simulink library "DAEMOT_Lib"  (R2019b)
settings: Solver=ode45  StartTime=0.0  StopTime=10.0  FixedStep=0.1  RelTol=1e-3
undefined symbols (not defined in the file or in its folder): Controller, CP, Ctrl, Ctrl_Fcn, Elec1, f, F2, Fluid, lag1, Mission, Moody, PropellerProp, rev_comms_sink
libraries: $bdroot x200, instrumentlib x21, simulink x5, dspsigops x2
(part 6 of 13)

== system DAEMOT_Lib/Thermal ==
  Air Volume : Subsystem  mask(Air volume){fld=Air, T_init=22, M_init=262.8177, P_init=105, Tamb_init=22, H=0, D=3, L=30, V=212.0575, A_sa=282.7433, Pamb=101, E_fluid=101*1e3}
      mask prompts: fld "Fluid Type"; T_init "Initial Air Temperature [°C]"; M_init "Initial Fluid Mass [kg]"; P_init "Air Pressure [kPa]"; Tamb_init "Initial Ambient Temperature [°C]"; H "Heat Transfer Coefficient with Ambient [W/m²K]"; D "Air Volume Diameter [m]"; L "Air Volume Length [m]"; V "Air Volume [m³]"; A_sa "Air Volume Surface Area [m²]"; Pamb "Ambient Pressure [kPa]"; E_fluid "Bulk Modulus"
      mask help: Tracks the time rate of change for fluid mass and temperature.
      mask init:
      | load('Fluids.mat');
      | Fluid = eval(['Fluid.',fld]);
      | 
      | % calculate the volume -- assuming a cylinder
      | V = L*pi*D^2/4;    
      | set_param(gcb,'V',num2str(V));
      | 
      | % calculate the surface area -- assuming a cylinder
      | SA = L * pi * D ;
      | set_param(gcb,'A_sa',num2str(SA));
      | 
      | % Note: Assumes a fixed initial pressure to calculate density
      | P_for_rho = 105;
      | Rho = qminterp2(Fluid.T, Fluid.P, Fluid.Rho_pt, T_init, P_for_rho);
      | 
      | % set the mass of air in the air volume
      | set_param(gcb,'M_init',num2str(Rho*V));
      settings: OpenFcn=|
      | load('Fluids.mat');
      | Set_Fluid_Popup_Names( Fluid )
      mask TypeOptions fld: Fuel | Water | Air | PG50
      mask DialogControl Container8 Prompt: Parameters
      mask DialogControl Container10 Prompt: Nonlinear Model
      mask DialogControl NomValuesGroupVar Prompt: Component Sizing - Nominal Values
      mask DialogControl Container11 Prompt: Linear Model
      mask Display:
      | image(imread('cabin.png'))
      | 
      | text(0.5,0.9,['{\bf Air Volume}'],'TexMode','on','horizontalAlignment', 'center')
      | text(0.5,0.1,['{(P)}'],'TexMode','on','horizontalAlignment', 'center')
      | 
      | port_label('input',1,'Flow In')
      | port_label('input',2,'Amb. Temp. [°C]')
      | port_label('input',3,'Q internal [kW]')
      | port_label('output',1,'Flow Out')
      | % port_label('output',2,'Fluid Mass [kg]')
  Cold_Plate : Subsystem  mask(Cold Plate){fld=PG50, P_init=113, Tw_init=20, T_init=20, f=0.035, KL=0, PAF=1, HTC_method=on, HTC=4000, M_wall=1, Cp_wall=0.9, D=0.03, L=1.5, t=0.0015, E=2.4e6, v=0.4, dH=0, e_rough=CP.e*1e-3}
      mask prompts: fld "Fluid Type"; P_init "Initial Outlet Pressure [kPa]"; Tw_init "Initial Wall Temperature [°C]"; T_init "Initial Outlet Temperature [°C]"; f "Friction Factor [-]"; KL "Minor Losses [-]"; PAF "HTC Parameter Adjustment Factor [-]"; HTC_method "User-Defined Heat Transfer Coefficient?"; HTC "Heat Transfer Coefficient [W/m^2*K]"; M_wall "Wall Mass [kg]"; Cp_wall "Wall Specific Heat [kJ/kg*K]"; D "Internal Diameter [m]"; L "Tube Length [m]"; t "Tube Wall Thickness [m]"; E "Tube Modulus of Elasticity [kPa]"; v "Tube Poisson Ratio [-]"; dH "Height between Inlet and Outlet [m]"; e_rough "Surface Roughness [m] (0.0015mm for copper, 0.01mm for rubber, 0mm for plastic)"
      mask help: Tracks the time rate of change of the pressure, wall temperature, and fluid exit temperature.
      mask init:
      | load('Fluids.mat');
      | Fluid = eval(['Fluid.',fld]);
      | 
      | load('Moody.mat');
      settings: OpenFcn=|
      | load('Fluids.mat');
      | Set_Fluid_Popup_Names( Fluid )
      mask TypeOptions fld: Fuel | Water | Air | PG50
      mask Callback HTC_method:
      | en = get_param(gcb,'MaskVisibilities');
      | 
      | switch get_param(gcb,'HTC_method')
      |     case 'on'
      |         en{9} = 'on';
      |     case 'off'
      |         en{9} = 'off';
      | end
      | set_param(gcb,'MaskVisibilities',en);
      mask DialogControl Container5 Prompt: Parameters
      mask DialogControl Container8 Prompt: Nonlinear Model
      mask DialogControl Container13 Prompt: Component Sizing - Nominal Values
      mask DialogControl Container11 Prompt: Linear Model
      mask Display:
      | image(imread('ColdPlate.jpg'))
      | 
      | text(0.5,0.95,['{\bf ',fld,' Cold Plate}'],'TexMode','on','horizontalAlignment', 'center')
      | text(0.5,0.08,['{-----(P)}'],'TexMode','on','horizontalAlignment', 'center')
      | 
      | port_label('input',1,'Flow In')
      | port_label('input',2,'Thermal In')
      | port_label('output',1,'Flow Out')
  Flow Split_Junction : Subsystem  mask(Split/Junction){fld=PG50, Num_Out=1, Num_In=1, P_init=110, T_init=22, D=0.013, L=0.1, t=0.0015, E=2.4e6, v=0.4}
      mask prompts: fld "Fluid Type"; Num_Out "Number of Outlet Flows"; Num_In "Number of Inlet Flows"; P_init "Initial Pressure [kPa]"; T_init "Initial Temperature [°C]"; D "Diameter [m]"; L "Length [m]"; t "Tube Wall Thickness [m]"; E "Tube Modulus of Elasticity [kPa]"; v "Tube Poisson Ratio [-]"
      mask help: Splits and junctions flows using dynamic relationships. Note that the library link of the block is disabled when it is imported into a model.
      mask init:
      | h      = get_param(gcb,'handle');   % Get block handle
      | blk    = gcb;
      | hblock = get(h);     % Parse out handles structure
      | 
      | load('Fluids.mat');
      | Fluid = eval(['Fluid.',fld]);
      | 
      | % delete any previous inports and bus selectors
      | for i = str2num(hblock.Num_In)+1:hblock.Ports(1)
      |     delete_block([blk,'/In',num2str(i)])
      |     delete_block([blk,'/gb',num2str(i)])
      |     delete_block([blk,'/gm',num2str(i)])
      |     delete_block([blk,'/gt',num2str(i)])
      |     delete_block([blk,'/gp',num2str(i)])
      |     delete_block([blk,'/Sink',num2str(i)])
      |     delete_block([blk,'/pout',num2str(i)])
      |     delete_block([blk,'/min',num2str(i)])
      |     delete_block([blk,'/tin',num2str(i)])
      |     
      |     delete_unconnected_lines(blk)
      | end
      | 
      | % delete any previous inports and bus selectors
      | for i = str2num(hblock.Num_Out)+1:hblock.Ports(2)
      |     delete_block([blk,'/Out',num2str(i)])
      |     delete_block([blk,'/m',num2str(i)])
      |     delete_block([blk,'/t',num2str(i)])
      |     delete_block([blk,'/p',num2str(i)])
      |     delete_block([blk,'/b',num2str(i)])
      |     delete_block([blk,'/Source',num2str(i)])
      |     delete_block([blk,'/g',num2str(i)])
      |     delete_block([blk,'/mout',num2str(i)])
      |     %delete_block([blk,'/tout',num2str(i)])
      |     
      |     delete_unconnected_lines(blk)
      | end
      | 
      | set_param([blk,'/Mux_In_1'],'Inputs',hblock.Num_In)
      | set_param([blk,'/Mux_In_2'],'Inputs',hblock.Num_Out)
      | set_param([blk,'/Mux_In_3'],'Inputs',hblock.Num_In)
      | %set_param([blk,'/Mux_Out_1'],'Outputs',hblock.Num_Out)
      | 
      | % generate inports, bus selectors, and route lines to each vector concat
      | for i = hblock.Ports(1)+1:str2num(hblock.Num_In)
      |     
      |     % add blocks
      |     add_block('simulink/Ports & Subsystems/In1',   [blk,'/In',num2str(i)],    'Position',[120 i*80-25+20 150 i*80-12+20]);         % adding inport
      |     add_block([blk,'/gb1'],                        [blk,'/gb',num2str(i)],   'Position',[200 i*80-20+20-18 205 i*80-2+20+2]);         % adding inport
      |     add_block('simulink/Signal Routing/Goto',      [blk,'/gm',num2str(i)],    'Position',[260 i*80-17 340 i*80-3]);         % adding inport
      |     add_block('simulink/Signal Routing/Goto',      [blk,'/gt',num2str(i)],    'Position',[260 i*80+3 340 i*80+17]);         % adding inport
      |     add_block('simulink/Sinks/Terminator',          [blk,'/gp',num2str(i)],    'Position',[260 i*80+23 280 i*80+37]);         % adding inport
      |     add_block('DAEMOT_Lib/Support Functions/Sink',[blk,'/Sink',num2str(i)],'Position',[745 i*80-14 810 i*80+14]);         % adding inport
      |     add_block('simulink/Signal Routing/From',      [blk,'/pout',num2str(i)],    'Position',[625 i*80-14 705 i*80+14]);         % adding inport
      |     add_block('simulink/Signal Routing/From',       [blk,'/min',num2str(i)],     'Position',[935 -258+i*20 1015 -242+i*20]);         % adding inport
      |     add_block('simulink/Signal Routing/From',       [blk,'/tin',num2str(i)],     'Position',[935 1+i*20 1015 19+i*20]);         % adding inport
      |     
      |     % set goto and from tags
      |     set_param([blk,'/gm',num2str(i)],'GotoTag',char(horzcat('M_in',num2str(i))))
      |     set_param([blk,'/gt',num2str(i)],'GotoTag',char(horzcat('T_in',num2str(i))))
      |     %set_param([blk,'/gp',num2str(i)],'GotoTag',char(horzcat('P_in',num2str(i))))
      |     set_param([blk,'/pout',num2str(i)],'GotoTag',char('P'))
      |     set_param([blk,'/min',num2str(i)],'GotoTag',char(horzcat('M_in',num2str(i))))
      |     set_param([blk,'/tin',num2str(i)],'GotoTag',char(horzcat('T_in',num2str(i))))
      |     
      |     % set goto and from background colors
      |     set_param([blk,'/gm',num2str(i)],'BackgroundColor','yellow')
      |     set_param([blk,'/gt',num2str(i)],'BackgroundColor','yellow')
      |     %set_param([blk,'/gp',num2str(i)],'BackgroundColor','yellow')
      |     set_param([blk,'/min',num2str(i)],'BackgroundColor','yellow')
      |     set_param([blk,'/tin',num2str(i)],'BackgroundColor','yellow')
      |     set_param([blk,'/pout',num2str(i)],'BackgroundColor','cyan')
      |     
      |     % add lines
      |     add_line(blk,['In',num2str(i),'/1'], ['gb',num2str(i),'/1'],'AutoRouting','on')
      |     add_line(blk,['gb',num2str(i),'/1'],  ['gm',num2str(i),'/1'],'AutoRouting','on')
      |     add_line(blk,['gb',num2str(i),'/2'],  ['gt',num2str(i),'/1'],'AutoRouting','on')
      |     add_line(blk,['gb',num2str(i),'/3'],  ['gp',num2str(i),'/1'],'AutoRouting','on')
      |     add_line(blk,['pout',num2str(i),'/1'],  ['Sink',num2str(i),'/1'],'AutoRouting','on')
      |     add_line(blk,['min',num2str(i),'/1'],  ['Mux_In_1/',num2str(i)],'AutoRouting','on')
      |     add_line(blk,['tin',num2str(i),'/1'],  ['Mux_In_3/',num2str(i)],'AutoRouting','on')
      |     
      | end
      | 
      | % generate inports, bus selectors, and route lines to each vector concat
      | for i = hblock.Ports(2)+1:str2num(hblock.Num_Out)
      |     
      |     % add blocks
      |     add_block('simulink/Ports & Subsystems/Out1',   [blk,'/Out',num2str(i)],   'Position',[30 i*80-25+20 60 i*80-12+20]);         % adding inport
      |     add_block('simulink/Signal Routing/From',       [blk,'/m',num2str(i)],     'Position',[-150 i*80-20 -70 i*80-2]);         % adding inport
      |     add_block('simulink/Signal Routing/From',       [blk,'/t',num2str(i)],     'Position',[-150 i*80-20+20 -70 i*80-2+20]);         % adding inport
      |     add_block('simulink/Signal Routing/From',       [blk,'/p',num2str(i)],     'Position',[-150 i*80-20+40 -70 i*80-2+40]);         % adding inport
      |     add_block('simulink/Signal Routing/Bus Creator',[blk,'/b',num2str(i)],     'Position',[5 i*80-20+20-18 10 i*80-2+20+2]);         % adding inport
      |     add_block('DAEMOT_Lib/Support Functions/Source',[blk,'/Source',num2str(i)],'Position',[395 i*80-14 460 i*80+14]);         % adding inport
      |     add_block('simulink/Signal Routing/Goto',       [blk,'/g',num2str(i)],     'Position',[505 i*80-9 585 i*80+9]);         % adding inport
      |     add_block('simulink/Signal Routing/From',       [blk,'/mout',num2str(i)],  'Position',[935 -129+i*20 1015 -111+i*20]);         % adding inport
      |     %add_block('simulink/Signal Routing/Goto',      [blk,'/tout',num2str(i)],   'Position',[1455 -259+i*20 1535 -241+i*20]);         % adding inport
      |     
      |     % set goto and from tags
      |     set_param([blk,'/m',num2str(i)],'GotoTag',char(horzcat('M_out',num2str(i))))
      |     %set_param([blk,'/t',num2str(i)],'GotoTag',char(horzcat('T_out',num2str(i))))
      |     set_param([blk,'/t',num2str(i)],'GotoTag',char('T'))
      |     set_param([blk,'/p',num2str(i)],'GotoTag',char('P'))
      |     set_param([blk,'/g',num2str(i)],'GotoTag',char(horzcat('M_out',num2str(i))))
      |     set_param([blk,'/mout',num2str(i)],'GotoTag',char(horzcat('M_out',num2str(i))))
      |     %set_param([blk,'/tout',num2str(i)],'GotoTag',char(horzcat('T_out',num2str(i))))
      |     set_param([blk,'/b',num2str(i)],'Inputs','3')
      |     
      |     % set goto and from background colors
      |     set_param([blk,'/t',num2str(i)],'BackgroundColor','cyan')
      |     set_param([blk,'/m',num2str(i)],'BackgroundColor','cyan')
      |     set_param([blk,'/p',num2str(i)],'BackgroundColor','cyan')
      |     set_param([blk,'/g',num2str(i)],'BackgroundColor','cyan')
      |     set_param([blk,'/mout',num2str(i)],'BackgroundColor','cyan')
      |     %set_param([blk,'/tout',num2str(i)],'BackgroundColor','cyan')
      |     
      |     % add lines
      |     add_line(blk,['m',num2str(i),'/1'],['b',num2str(i),'/1'],'AutoRouting','on')
      |     p = get_param([blk,'/m',num2str(i)],'PortHandles');
      |     l = get_param(p.Outport,'Line');
      |     set_param(l,'Name','mdot_kgps')
      |     
      |     add_line(blk,['t',num2str(i),'/1'],['b',num2str(i),'/2'],'AutoRouting','on')
      |     p = get_param([blk,'/t',num2str(i)],'PortHandles');
      |     l = get_param(p.Outport,'Line');
      |     set_param(l,'Name','T_C')
      |     
      |     add_line(blk,['p',num2str(i),'/1'],['b',num2str(i),'/3'],'AutoRouting','on')
      |     p = get_param([blk,'/p',num2str(i)],'PortHandles');
      |     l = get_param(p.Outport,'Line');
      |     set_param(l,'Name','P_kPa')
      |     
      |     add_line(blk,['b',num2str(i),'/1'],['Out',num2str(i),'/1'],'AutoRouting','on')
      |     add_line(blk,['Source',num2str(i),'/1'],['g',num2str(i),'/1'],'AutoRouting','on')
      |     add_line(blk,['mout',num2str(i),'/1'],  ['Mux_In_2/',num2str(i)],'AutoRouting','on')
      |     %add_line(blk,['Mux_Out_1/',num2str(i)], ['tout',num2str(i),'/1'],'AutoRouting','on')
      | end
      | 
      | try
      |     set_param([blk,'/Selector1'],'InputPortWidth',num2str(hblock.Num_In))
      |     set_param([blk,'/Selector2'],'InputPortWidth',num2str(hblock.Num_In))
      |     
      |     selector_str = '[1 ';
      |     for i = 2:str2num(hblock.Num_In)
      |         selector_str = [selector_str,num2str(i),' '];
      |     end
      |     selector_str = [selector_str,']'];
      |     set_param([blk,'/Selector1'],'IndexParamArray',{selector_str})%num2cell(1:hblock.Num_In))
      |     set_param([blk,'/Selector2'],'IndexParamArray',{selector_str})%num2cell(1:hblock.Num_In))
      | catch
      |     selector_str = '[1 ';
      |     for i = 2:str2num(hblock.Num_In)
      |         selector_str = [selector_str,num2str(i),' '];
      |     end
      |     selector_str = [selector_str,']'];
      |     set_param([blk,'/Selector1'],'IndexParamArray',{selector_str})%num2cell(1:hblock.Num_In))
      |     set_param([blk,'/Selector2'],'IndexParamArray',{selector_str})%num2cell(1:hblock.Num_In))
      |     
      |     set_param([blk,'/Selector1'],'InputPortWidth',num2str(hblock.Num_In))
      |     set_param([blk,'/Selector2'],'InputPortWidth',num2str(hblock.Num_In))
      | end 
      |     
      |     clear h blk hblock
      settings: CopyFcn=|
      | h      = get_param(gcb,'handle');   % Get block handle
      | blk    = gcb;
      | 
      | set_param(blk, 'LinkStatus', 'inactive')
      settings: OpenFcn=|
      | load('Fluids.mat');
      | Set_Fluid_Popup_Names( Fluid )
      mask TypeOptions fld: Fuel | Water | Air | PG50
      mask DialogControl Container4 Prompt: Parameters
      mask DialogControl Container12 Prompt: Nonlinear Model
      mask DialogControl Container15 Prompt: Component Sizing - Nominal Values
      mask Display:
      | image(imread('Split.jpg'));
      | 
      | text(0.5,0.95,['{\bf',fld,' Split/Junction}'],'TexMode','on','horizontalAlignment', 'center')
      | text(0.5,0.08,['{(P)}'],'TexMode','on','horizontalAlignment', 'center')
      | 
      | h      = get_param(gcb,'handle');   % Get block handle
      | blk    = gcb;
      | hblock = get(h);     % Parse out handles structure
      | for i = 1:str2num(hblock.Num_In)
      |     port_label('input',i,horzcat('Flow In #',num2str(i)))
      | end
      | for i = 1:str2num(hblock.Num_Out)
      |     port_label('output',i,horzcat('Flow Out #',num2str(i)))
      | end
  Heat Exchanger : Subsystem  mask(Heat Exchanger){Tw_init=22, fld1=PG50, P1_init=110, T1_init=22, f1=0.05, KL1=0, HTC_method1=on, HTC1=2.5715e+03, fld2=PG50, P2_init=110, T2_init=22, f2=0.05, KL2=0, HTC_method2=on, HTC2=2.5715e+03, M_wall=0.1, Cp_wall=0.9, Pass1=6, b1=1*1e-3, W1=87*1e-3, L1=0.193, dH1=0.193, e1=0.0015*1e-3, Nu_lam1=5.6153, Pass2=6, b2=1*1e-3, W2=87*1e-3, L2=0.193, dH2=-0.193, e2=0.0015*1e-3, Nu_lam2=5.6153}
      mask prompts: Tw_init "Initial Wall Temperature [°C]"; fld1 "Fluid Type 1"; P1_init "Initial Outlet 1 Pressure [kPa]"; T1_init "Initial Outlet 1 Temperature [°C]"; f1 "Friction Factor [-]"; KL1 "Minor Losses [-]"; HTC_method1 "User-Defined Heat Transfer Coefficient?"; HTC1 "Heat Transfer Coefficient [W/m^2*K]"; fld2 "Fluid Type 2"; P2_init "Initial Outlet 2 Pressure [kPa]"; T2_init "Initial Outlet 2 Temperature [°C]"; f2 "Friction Factor [-]"; KL2 "Minor Losses [-]"; HTC_method2 "User-Defined Heat Transfer Coefficient?"; HTC2 "Heat Transfer Coefficient [W/m^2*K]"; M_wall "Single Wall Mass [kg]"; Cp_wall "Wall Specific Heat [kJ/kg*K]"; Pass1 "Number of Passes"; b1 "Plate Spacing [m]"; W1 "Plate Width [m]"; L1 "Plate Length [m]"; dH1 "Height between Inlet and Outlet [m]"; e1 "Surface Roughness [m] (0.0015mm for copper, 0.01mm for rubber, 0mm for plastic)"; Nu_lam1 "Laminar Nu"; Pass2 "Number of Passes"; b2 "Plate Spacing [m]"; W2 "Plate Width [m]"; L2 "Plate Length [m]"; dH2 "Height between Inlet and Outlet [m]"; e2 "Surface Roughness [m] (0.0015mm for copper, 0.01mm for rubber, 0mm for plastic)"; Nu_lam2 "Laminar Nu"
      mask help: Tracks the time rate of change of the pressure, wall temperature, and exit flow temperatures.
      mask init:
      | load('Fluids.mat');
      | Fluid1 = eval(['Fluid.',fld1]);
      | Fluid2 = eval(['Fluid.',fld2]);
      | 
      | load('Moody.mat');
      | 
      | load('Laminar_Props.mat')
      | Nu_lam1 = interp1(LamProps.b_a,LamProps.Nu,max(W1,b1)/min(W1,b1));
      | Nu_lam2 = interp1(LamProps.b_a,LamProps.Nu,max(W2,b2)/min(W2,b2));
      | set_param(gcb,'Nu_lam1',num2str(Nu_lam1));
      | set_param(gcb,'Nu_lam2',num2str(Nu_lam2));
      settings: OpenFcn=|
      | load('Fluids.mat');
      | Set_Fluid_Popup_Names( Fluid )
      mask TypeOptions fld1: Fuel | Water | Air | PG50
      mask Callback HTC_method1:
      | en = get_param(gcb,'MaskVisibilities');
      | 
      | switch get_param(gcb,'HTC_method1')
      |     case 'on'
      |         en{8} = 'on';
      |     case 'off'
      |         en{8} = 'off';
      | end
      | set_param(gcb,'MaskVisibilities',en);
      mask TypeOptions fld2: Fuel | Water | Air | PG50
      mask Callback HTC_method2:
      | en = get_param(gcb,'MaskVisibilities');
      | 
      | switch get_param(gcb,'HTC_method2')
      |     case 'on'
      |         en{16} = 'on';
      |     case 'off'
      |         en{16} = 'off';
      | end
      | set_param(gcb,'MaskVisibilities',en);
      mask DialogControl Container10 Prompt: Parameters
      mask DialogControl Container18 Prompt: Side 1
      mask DialogControl Container17 Prompt: Side 2
      mask DialogControl Container7 Prompt: Nonlinear Model
      mask DialogControl Container14 Prompt: Component Sizing - Nominal Values
      mask DialogControl Container8 Prompt: Side 1
      mask DialogControl Container9 Prompt: Side 2
      mask DialogControl Container6 Prompt: Linear Model
      mask Display:
      | image(imread('HX.jpg'))
      | 
      | text(0.5,0.95,['{\bf ',fld1,'/',fld2,' HX}'],'TexMode','on','horizontalAlignment', 'center')
      | text(0.5,0.08,['{-----(P)}'],'TexMode','on','horizontalAlignment', 'center')
      | 
      | port_label('input',1,['In 1 (',fld1,')'])
      | port_label('input',2,['In 2 (',fld2,')'])
      | port_label('output',1,['Out 1 (',fld1,')'])
      | port_label('output',2,['Out 2 (',fld2,')'])
  Heat_Sink_Edge : Subsystem  mask(Heat Sink Edge){s=off, R_const=1, k=237, As=.025, L=.02}
      mask prompts: s "Constant Resistance"; R_const "Plate Resistance [K/W]"; k "Thermal Conductivity [W/m-K]"; As "Surface Area [m^2]"; L "Plate Thickness [m]"
      mask help: Computes the rate of convective heat transfer between two temperature elements.
      mask Callback s:
      | str = get_param(gcb,'s');
      | me = get_param(gcb,'MaskEnables');
      | 
      | switch str
      |     case 'on'
      |         me{2} = 'on';
      |         me{3} = 'off';
      |         me{4} = 'off';
      |         me{5} = 'off';
      |     case 'off'
      |         me{2} = 'off';
      |         me{3} = 'on';
      |         me{4} = 'on';
      |         me{5} = 'on';
      | end
      | set_param(gcb,'MaskEnables',me);
      mask DialogControl ParameterTabVar0 Prompt: Cooling Parameters
      mask DialogControl ParameterTabVar012 Prompt: System
      mask Display:
      | % image(imread('inductor.bmp'));
      | text(0.5,0.95,['{\bf Heat Sink Edge}'],'TexMode','on','horizontalAlignment', 'center')
      | text(0.5,0.075,['{\bf ----}'],'TexMode','on','horizontalAlignment', 'center')
      | 
      | port_label('input',1,sprintf('Thermal \nIn'))
      | 
      | port_label('output',1,sprintf('Thermal \nOut'))
  Multi-Port Fluid Tank : Subsystem  mask(Multi-Port Fluid Tank){fld=PG50, Num_Out=2, Num_In=2, T_init=22, h_init=0.2, M_init=1.0433, P_init=103.0361, Tamb_init=22, H=0, D=0.08, Pamb=101}
      mask prompts: fld "Fluid Type"; Num_Out "Number of Outlet Flows"; Num_In "Number of Inlet Flows"; T_init "Initial Fluid Temperature [°C]"; h_init "Initial Fluid Height [m]"; M_init "Initial Fluid Mass [kg] (fcn of height)"; P_init "Initial Fluid Pressure [kPa] (fcn of height)"; Tamb_init "Initial Ambient Temperature [°C]"; H "Heat Transfer Coefficient [W/m²K]"; D "Tank Diameter [m]"; Pamb "Ambient Pressure [kPa]"
      mask help: Tracks the time rate of change for fluid mass and temperature, allowing for multiple inlet and outlet flows.
      mask init:
      | h      = get_param(gcb,'handle');   % Get block handle
      | blk    = gcb;
      | hblock = get(h);     % Parse out handles structure
      | 
      | load('Fluids.mat');
      | Fluid = eval(['Fluid.',fld]);
      | 
      | % Note: Assumes a fixed initial pressure to calculate density
      | P_for_rho = 105;
      | Rho = qminterp2(Fluid.T, Fluid.P, Fluid.Rho_pt, T_init, P_for_rho);
      | 
      | M_init = h_init*Rho*pi*D^2/4;
      | set_param(gcb,'M_init',num2str(M_init));
      | 
      | P_init = Rho*9.81*h_init/1000 + Pamb;
      | set_param(gcb,'P_init',num2str(P_init));
      | 
      | % delete any previous inports and bus selectors
      | for i = str2num(hblock.Num_In)+1:hblock.Ports(1)-1
      |     delete_block([blk,'/In',num2str(i)])
      |     delete_block([blk,'/gb',num2str(i)])
      |     delete_block([blk,'/gm',num2str(i)])
      |     delete_block([blk,'/gt',num2str(i)])
      |     delete_block([blk,'/gp',num2str(i)])
      |     delete_block([blk,'/Sink',num2str(i)])
      |     delete_block([blk,'/pout',num2str(i)])
      |     delete_block([blk,'/min',num2str(i)])
      |     delete_block([blk,'/tin',num2str(i)])
      |     
      |     delete_unconnected_lines(blk)
      | end
      | 
      | % delete any previous inports and bus selectors
      | for i = str2num(hblock.Num_Out)+1:hblock.Ports(2)
      |     delete_block([blk,'/Out',num2str(i)])
      |     delete_block([blk,'/m',num2str(i)])
      |     delete_block([blk,'/t',num2str(i)])
      |     delete_block([blk,'/p',num2str(i)])
      |     delete_block([blk,'/b',num2str(i)])
      |     delete_block([blk,'/Source',num2str(i)])
      |     delete_block([blk,'/g',num2str(i)])
      |     delete_block([blk,'/mout',num2str(i)])
      |     %delete_block([blk,'/tout',num2str(i)])
      |     
      |     delete_unconnected_lines(blk)
      | end
      | 
      | set_param([blk,'/Mux_In_1'],'Inputs',hblock.Num_In)
      | set_param([blk,'/Mux_In_2'],'Inputs',hblock.Num_Out)
      | set_param([blk,'/Mux_In_3'],'Inputs',hblock.Num_In)
      | %set_param([blk,'/Mux_Out_1'],'Outputs',hblock.Num_Out)
      | 
      | % generate inports, bus selectors, and route lines to each vector concat
      | for i = hblock.Ports(1):str2num(hblock.Num_In)
      |     
      |     % add blocks
      |     add_block('simulink/Ports & Subsystems/In1',   [blk,'/In',num2str(i)],    'Position',[120 i*80-25+20 150 i*80-12+20]);         % adding inport
      |     add_block([blk,'/gb1'],                        [blk,'/gb',num2str(i)],   'Position',[200 i*80-20+20-18 205 i*80-2+20+2]);         % adding inport
      |     add_block('simulink/Signal Routing/Goto',      [blk,'/gm',num2str(i)],    'Position',[260 i*80-17 340 i*80-3]);         % adding inport
      |     add_block('simulink/Signal Routing/Goto',      [blk,'/gt',num2str(i)],    'Position',[260 i*80+3 340 i*80+17]);         % adding inport
      |     add_block('simulink/Sinks/Terminator',          [blk,'/gp',num2str(i)],    'Position',[260 i*80+23 280 i*80+37]);         % adding inport
      |     add_block('DAEMOT_Lib/Support Functions/Sink',[blk,'/Sink',num2str(i)],'Position',[745 i*80-14 810 i*80+14]);         % adding inport
      |     add_block('simulink/Signal Routing/From',      [blk,'/pout',num2str(i)],    'Position',[625 i*80-14 705 i*80+14]);         % adding inport
      |     add_block('simulink/Signal Routing/From',       [blk,'/min',num2str(i)],     'Position',[935 -258+i*20 1015 -242+i*20]);         % adding inport
      |     add_block('simulink/Signal Routing/From',       [blk,'/tin',num2str(i)],     'Position',[935 1+i*20 1015 19+i*20]);         % adding inport
      |     
      |     % set input port numbers
      |     set_param([blk,'/In',num2str(i)],'Port',num2str(i))
      |     
      |     % set goto and from tags
      |     set_param([blk,'/gm',num2str(i)],'GotoTag',char(horzcat('M_in',num2str(i))))
      |     set_param([blk,'/gt',num2str(i)],'GotoTag',char(horzcat('T_in',num2str(i))))
      |     %set_param([blk,'/gp',num2str(i)],'GotoTag',char(horzcat('P_in',num2str(i))))
      |     set_param([blk,'/pout',num2str(i)],'GotoTag',char('P_tank'))
      |     set_param([blk,'/min',num2str(i)],'GotoTag',char(horzcat('M_in',num2str(i))))
      |     set_param([blk,'/tin',num2str(i)],'GotoTag',char(horzcat('T_in',num2str(i))))
      |     
      |     % set goto and from background colors
      |     set_param([blk,'/gm',num2str(i)],'BackgroundColor','yellow')
      |     set_param([blk,'/gt',num2str(i)],'BackgroundColor','yellow')
      |     %set_param([blk,'/gp',num2str(i)],'BackgroundColor','yellow')
      |     set_param([blk,'/min',num2str(i)],'BackgroundColor','yellow')
      |     set_param([blk,'/tin',num2str(i)],'BackgroundColor','yellow')
      |     set_param([blk,'/pout',num2str(i)],'BackgroundColor','cyan')
      |     
      |     % add lines
      |     add_line(blk,['In',num2str(i),'/1'], ['gb',num2str(i),'/1'],'AutoRouting','on')
      |     add_line(blk,['gb',num2str(i),'/1'],  ['gm',num2str(i),'/1'],'AutoRouting','on')
      |     add_line(blk,['gb',num2str(i),'/2'],  ['gt',num2str(i),'/1'],'AutoRouting','on')
      |     add_line(blk,['gb',num2str(i),'/3'],  ['gp',num2str(i),'/1'],'AutoRouting','on')
      |     add_line(blk,['pout',num2str(i),'/1'],  ['Sink',num2str(i),'/1'],'AutoRouting','on')
      |     add_line(blk,['min',num2str(i),'/1'],  ['Mux_In_1/',num2str(i)],'AutoRouting','on')
      |     add_line(blk,['tin',num2str(i),'/1'],  ['Mux_In_3/',num2str(i)],'AutoRouting','on')
      |     
      | end
      | 
      | % generate inports, bus selectors, and route lines to each vector concat
      | for i = hblock.Ports(2)+1:str2num(hblock.Num_Out)
      |     
      |     % add blocks
      |     add_block('simulink/Ports & Subsystems/Out1',   [blk,'/Out',num2str(i)],   'Position',[30 i*80-25+20 60 i*80-12+20]);         % adding inport
      |     add_block('simulink/Signal Routing/From',       [blk,'/m',num2str(i)],     'Position',[-150 i*80-20 -70 i*80-2]);         % adding inport
      |     add_block('simulink/Signal Routing/From',       [blk,'/t',num2str(i)],     'Position',[-150 i*80-20+20 -70 i*80-2+20]);         % adding inport
      |     add_block('simulink/Signal Routing/From',       [blk,'/p',num2str(i)],     'Position',[-150 i*80-20+40 -70 i*80-2+40]);         % adding inport
      |     add_block('simulink/Signal Routing/Bus Creator',[blk,'/b',num2str(i)],     'Position',[5 i*80-20+20-18 10 i*80-2+20+2]);         % adding inport
      |     add_block('DAEMOT_Lib/Support Functions/Source',[blk,'/Source',num2str(i)],'Position',[395 i*80-14 460 i*80+14]);         % adding inport
      |     add_block('simulink/Signal Routing/Goto',       [blk,'/g',num2str(i)],     'Position',[505 i*80-9 585 i*80+9]);         % adding inport
      |     add_block('simulink/Signal Routing/From',       [blk,'/mout',num2str(i)],  'Position',[935 -129+i*20 1015 -111+i*20]);         % adding inport
      |     %add_block('simulink/Signal Routing/Goto',      [blk,'/tout',num2str(i)],   'Position',[1455 -259+i*20 1535 -241+i*20]);         % adding inport
      |     
      |     % set goto and from tags
      |     set_param([blk,'/m',num2str(i)],'GotoTag',char(horzcat('M_out',num2str(i))))
      |     %set_param([blk,'/t',num2str(i)],'GotoTag',char(horzcat('T_out',num2str(i))))
      |     set_param([blk,'/t',num2str(i)],'GotoTag',char('T_tank'))
      |     set_param([blk,'/p',num2str(i)],'GotoTag',char('P_tank'))
      |     set_param([blk,'/g',num2str(i)],'GotoTag',char(horzcat('M_out',num2str(i))))
      |     set_param([blk,'/mout',num2str(i)],'GotoTag',char(horzcat('M_out',num2str(i))))
      |     %set_param([blk,'/tout',num2str(i)],'GotoTag',char(horzcat('T_out',num2str(i))))
      |     set_param([blk,'/b',num2str(i)],'Inputs','3')
      |     
      |     % set goto and from background colors
      |     set_param([blk,'/t',num2str(i)],'BackgroundColor','cyan')
      |     set_param([blk,'/m',num2str(i)],'BackgroundColor','cyan')
      |     set_param([blk,'/p',num2str(i)],'BackgroundColor','cyan')
      |     set_param([blk,'/g',num2str(i)],'BackgroundColor','cyan')
      |     set_param([blk,'/mout',num2str(i)],'BackgroundColor','cyan')
      |     %set_param([blk,'/tout',num2str(i)],'BackgroundColor','cyan')
      |     
      |     % add lines
      |     add_line(blk,['m',num2str(i),'/1'],['b',num2str(i),'/1'],'AutoRouting','on')
      |     p = get_param([blk,'/m',num2str(i)],'PortHandles');
      |     l = get_param(p.Outport,'Line');
      |     set_param(l,'Name','mdot_kgps')
      |     
      |     add_line(blk,['t',num2str(i),'/1'],['b',num2str(i),'/2'],'AutoRouting','on')
      |     p = get_param([blk,'/t',num2str(i)],'PortHandles');
      |     l = get_param(p.Outport,'Line');
      |     set_param(l,'Name','T_C')
      |     
      |     add_line(blk,['p',num2str(i),'/1'],['b',num2str(i),'/3'],'AutoRouting','on')
      |     p = get_param([blk,'/p',num2str(i)],'PortHandles');
      |     l = get_param(p.Outport,'Line');
      |     set_param(l,'Name','P_kPa')
      |     
      |     add_line(blk,['b',num2str(i),'/1'],['Out',num2str(i),'/1'],'AutoRouting','on')
      |     add_line(blk,['Source',num2str(i),'/1'],['g',num2str(i),'/1'],'AutoRouting','on')
      |     add_line(blk,['mout',num2str(i),'/1'],  ['Mux_In_2/',num2str(i)],'AutoRouting','on')
      |     %add_line(blk,['Mux_Out_1/',num2str(i)], ['tout',num2str(i),'/1'],'AutoRouting','on')
      | end
      | 
      | try
      |     set_param([blk,'/Selector1'],'InputPortWidth',num2str(hblock.Num_In))
      |     set_param([blk,'/Selector2'],'InputPortWidth',num2str(hblock.Num_In))
      |     
      |     selector_str = '[1 ';
      |     for i = 2:str2num(hblock.Num_In)
      |         selector_str = [selector_str,num2str(i),' '];
      |     end
      |     selector_str = [selector_str,']'];
      |     set_param([blk,'/Selector1'],'IndexParamArray',{selector_str})%num2cell(1:hblock.Num_In))
      |     set_param([blk,'/Selector2'],'IndexParamArray',{selector_str})%num2cell(1:hblock.Num_In))
      | catch
      |     selector_str = '[1 ';
      |     for i = 2:str2num(hblock.Num_In)
      |         selector_str = [selector_str,num2str(i),' '];
      |     end
      |     selector_str = [selector_str,']'];
      |     set_param([blk,'/Selector1'],'IndexParamArray',{selector_str})%num2cell(1:hblock.Num_In))
      |     set_param([blk,'/Selector2'],'IndexParamArray',{selector_str})%num2cell(1:hblock.Num_In))
      |     
      |     set_param([blk,'/Selector1'],'InputPortWidth',num2str(hblock.Num_In))
      |     set_param([blk,'/Selector2'],'InputPortWidth',num2str(hblock.Num_In))
      | end 
      |     
      |     clear h blk hblock
      settings: CopyFcn=|
      | h      = get_param(gcb,'handle');   % Get block handle
      | blk    = gcb;
      | 
      | set_param(blk, 'LinkStatus', 'inactive')
      settings: OpenFcn=|
      | load('Fluids.mat');
      | Set_Fluid_Popup_Names( Fluid )
      mask TypeOptions fld: Fuel | Water | Air | PG50
      mask DialogControl Container8 Prompt: Parameters
      mask DialogControl Container10 Prompt: Nonlinear Model
      mask DialogControl NomValuesGroupVar Prompt: Component Sizing - Nominal Values
      mask DialogControl Container11 Prompt: Linear Model
      mask Display:
      | image(imread('Res.jpg'))
      | 
      | text(0.5,0.95,['{\bf ',fld,' Multi-Port Tank}'],'TexMode','on','horizontalAlignment', 'center')
      | text(0.5,0.08,['{(P)}'],'TexMode','on','horizontalAlignment', 'center')
      | 
      | % port_label('input',1,'Flow In')
      | % port_label('input',2,'Amb. Temp. [°C]')
      | % port_label('output',1,'Flow Out')
      | 
      | h      = get_param(gcb,'handle');   % Get block handle
      | blk    = gcb;
      | hblock = get(h);     % Parse out handles structure
      | for i = 1:str2num(hblock.Num_In)
      |     port_label('input',i,horzcat('Flow In #',num2str(i)))
      | end
      | port_label('input',str2num(hblock.Num_In)+1,'Amb. Temp. [°C]')
      | for i = 1:str2num(hblock.Num_Out)
      |     port_label('output',i,horzcat('Flow Out #',num2str(i)))
      | end
  PCM Module : Subsystem  mask(PCM Module){hc_config=Stacked, heat sink on top, dim1=.75, dim2=.75, depth=.01, L=.75, t_h=.005, R_cont=1/11400, T_melt_ID=off, c_T_melt=30, por=1, H_ID=Aluminum, F_ID=Copper, PCM_ID=ParaffinWax, V_L_0=0, T_1_0=25}
      mask prompts: hc_config "Heat Sink/Component Config"; dim1 "Cross Section Dimension 1 (m)"; dim2 "Cross Section Dimension 2 (m)"; depth "Depth (m)"; L "Vertical Side Length (m)"; t_h "Housing Thickness (m)"; R_cont "Contact Resistance (m^2K/W)"; T_melt_ID "Custom T_melt?"; c_T_melt "T_melt (C)"; por "Porosity"; H_ID "Housing Material"; F_ID "Foam Material"; PCM_ID "Phase Change Material"; V_L_0 "Liquid Volume Fraction"; T_1_0 "Inner Surface Temperature (C)"
      mask help: Models a PCM Module.
      mask init:
      | load('PCMProps.mat');
      | L=str2double(L);
      | 
      | if strcmp(PCM_ID,'ParaffinWax')
      |     PCM_info=PCMProps.ParaffinWax;
      | elseif strcmp(PCM_ID,'nEicosane')
      |     PCM_info=PCMProps.nEicosane;
      | elseif strcmp(PCM_ID,'RT28HC')
      |     PCM_info=PCMProps.RT28HC;
      | end
      | 
      | k_l=PCM_info.Thermal_Conductivity;
      | L_pcm=PCM_info.Latent_heat;
      | rho_pcm=PCM_info.Density;
      | c_pcm=PCM_info.Specific_Heat;
      | beta=PCM_info.Volumetric_Thermal_Expansion_Coefficient;
      | nu=PCM_info.Kinematic_Viscosity;
      | switch T_melt_ID
      |     case logical(1)
      |     T_melt = c_T_melt;
      |     otherwise
      |     T_melt=PCM_info.Melt_temperature;
      | end
      | 
      | if strcmp(H_ID,'Aluminum')
      |     k_h=237;    %W/(mK)
      |     c_h=903; %J/(kgK)
      |     rho_h=2702; %kg/m^3
      | elseif strcmp(H_ID,'Copper')
      |     k_h=401;    %W/(mK)
      |     c_h=385;    %J/kgK
      |     rho_h=8933; %kg/m^3
      | end
      | 
      | if strcmp(F_ID,'Aluminum')
      |     k_f=237;    %W/(mK)
      |     c_f=903; %J/(kgK)
      |     rho_f=2702; %kg/m^3
      | elseif strcmp(F_ID,'Copper')
      |     k_f=401;    %W/(mK)
      |     c_f=385;    %J/kgK
      |     rho_f=8933; %kg/m^3
      | end
      | 
      | 
      | 
      | if V_L_0==0
      |     V_L_0=1e-5;
      | end
      | 
      | if strcmp(hc_config,'Side-by-side')
      |     hc_config=1;
      | elseif strcmp(hc_config,'Stacked, heat sink on top')
      |     hc_config=2;
      | elseif strcmp(hc_config,'Stacked, heat sink on bottom')
      |     hc_config=3;
      | end
      mask TypeOptions hc_config: Side-by-side | Stacked, heat sink on top | Stacked, heat sink on bottom
      mask Callback hc_config:
      | en=get_param(gcb,'MaskEnables');
      | switch get_param(gcb,'hc_config')
      |     case 'Side-by-side'
      |         en{5}='on';
      |     otherwise
      |         en{5}='off';
      | end
      | set_param(gcb,'MaskEnables',en);
      mask Callback dim1:
      | ms=get_param(gcb,'MaskStyles');
      | dim1=get_param(gcb,'dim1');
      | dim2=get_param(gcb,'dim2');
      | ms{5}=['popup(',num2str(dim1),'|',num2str(dim2),')'];
      | set_param(gcb,'MaskStyles',ms);
      mask Callback dim2:
      | ms=get_param(gcb,'MaskStyles');
      | dim1=get_param(gcb,'dim1');
      | dim2=get_param(gcb,'dim2');
      | ms{5}=['popup(',num2str(dim1),'|',num2str(dim2),')'];
      | set_param(gcb,'MaskStyles',ms);
      mask TypeOptions L: .75 | .75
      mask Callback T_melt_ID:
      | en=get_param(gcb,'MaskEnables');
      | switch get_param(gcb,'T_melt_ID')
      |     case 'on'
      |         en{9}='on';
      |     otherwise
      |         en{9}='off';
      | end
      | set_param(gcb,'MaskEnables',en);
      mask TypeOptions H_ID: Aluminum | Copper
      mask TypeOptions F_ID: Copper | Aluminum
      mask TypeOptions PCM_ID: ParaffinWax | nEicosane | RT28HC
      mask DialogControl DescTextVar Prompt: Input desired heat sink properties. Heat sink assumed rectangular with constant housing thickness surrounding PCM.
      mask DialogControl Container6 Prompt: Parameters
      mask DialogControl Container12 Prompt: Initial Conditions
      mask Display:
      | image(imread('pcmheatsink.png'))
      | 
      | text(.5,.9,['{\bf PCM Module}'],'TexMode','on','horizontalAlignment', 'center')
      | 
      | port_label('input',1,sprintf('Cooling \nSide2'))
      | 
      | port_label('output',1,sprintf('Cooling \nSide1'))
  Peristaltic_Pump : Subsystem  mask(Peristaltic Pump){H_k=[-0.0003743 0.0001507 0.000003070]}
      mask prompts: H_k "Drain map coefficients [K PWM P]"
      mask help: Models a peristaltic pump as a function of upstream pressure and pump command.
      mask DialogControl ParameterGroupVar Prompt: Nonlinear Model
      mask Display:
      | image(imread('DrainPump.jpg'))
      | 
      | text(0.5, 0.95,['{\bf Peristaltic Pump}'],'TexMode','on','horizontalAlignment', 'center')
      | text(0.5,0.1,['{-----}'],'TexMode','on','horizontalAlignment', 'center')
      | 
      | port_label('input',1,'Flow In')
      | port_label('input',2,'Speed [0-10]')
      | port_label('output',1,'Flow Out')
      | port_label('output',2,'M_Out [kg/s]')
  Pipe_P_to_M : Subsystem  mask(Pipe (P to M)){fld=PG50, T_init=22, P_init=101, Tamb_init=22, f=0.05, KL_tube=0, KL=0, H=0, D=13*1e-3, L=0.1, t=0.0015, E=2.4e6, v=0.4, dH=0, e_rough=0.01*1e-3, Num_MFRS=0, Num_PS=0, Num_TS=0, Num_BV=0, Num_CV=0}
      mask prompts: fld "Fluid Type"; T_init "Initial Outlet Temperature [°C]"; P_init "Initial Outlet Pressure [kPa]"; Tamb_init "Initial Ambient Temperature [°C]"; f "Tube Friction Factor [-]"; KL_tube "Tube Minor Losses [-]"; KL "Total Minor Losses [-]"; H "Heat Transfer Coefficient [W/m²K]"; D "Pipe Internal Diameter [m]"; L "Pipe Length [m]"; t "Tube Wall Thickness [m]"; E "Tube Modulus of Elasticity [kPa]"; v "Tube Poisson Ratio [-]"; dH "Height between Inlet and Outlet [m]"; e_rough "Surface Roughness [m] (0.0015mm for copper, 0.01mm for rubber, 0mm for plastic)"; Num_MFRS "Number of Mass Flow Rate Sensors"; Num_PS "Number of Pressure Sensors"; Num_TS "Number of Temperature Sensors"; Num_BV "Number of Ball Valves"; Num_CV "Number of Check Valves"
      mask help: Models a pipe given an upstream pressure and downstream mass flow rate.
      mask init:
      | load('Fluids.mat');
      | Fluid = eval(['Fluid.',fld]);
      | 
      | load('Moody.mat');
      | 
      | KL = KL_correction(KL_tube,Num_MFRS,Num_PS,Num_TS,Num_BV,Num_CV);
      | set_param(gcb,'KL',num2str(KL));
      settings: OpenFcn=|
      | load('Fluids.mat');
      | Set_Fluid_Popup_Names( Fluid )
      mask TypeOptions fld: Fuel | Water | Air | PG50
      mask DialogControl Container8 Prompt: Parameters
      mask DialogControl Container10 Prompt: Nonlinear Model
      mask DialogControl NomValuesGroupVar Prompt: Component Sizing - Nominal Values
      mask DialogControl Container11 Prompt: Linear Model
      mask DialogControl Container16 Prompt: Sensors and Valves
      mask Display:
      | if sum([Num_MFRS,Num_PS,Num_TS,Num_BV,Num_CV])==0
      |     image(imread('Tube.jpg'))
      | elseif sum([Num_MFRS,Num_PS,Num_TS])~=0 && sum([Num_BV,Num_CV])==0
      |     image(imread('Tube_Sensor.jpg'))
      | elseif sum([Num_MFRS,Num_PS,Num_TS])==0 && sum([Num_BV,Num_CV])~=0
      |     image(imread('Tube_Valve.jpg'))
      | else
      |     image(imread('Tube_Valve_Sensor.jpg'))
      | end
      | 
      | text(0.5,0.95,['{\bf ',fld,' Pipe (P to M)}'],'TexMode','on','horizontalAlignment', 'center')
      | text(0.5,0.1,['{-----(P)}'],'TexMode','on','horizontalAlignment', 'center')
      | 
      | port_label('input',1,'Flow In')
      | port_label('input',2,'Amb. Temp. [°C]')
      | port_label('output',1,'Flow Out')
  Pipe_P_to_P : Subsystem  mask(Pipe (P to P)){fld=PG50, T_init=22, Tamb_init=22, f=0.05, KL_tube=0, KL=0, H=0, D=13*1e-3, L=0.1, t=0.0015, E=2.4e6, v=0.4, dH=0, e_rough=0.01*1e-3, Num_MFRS=0, Num_PS=0, Num_TS=0, Num_BV=0, Num_CV=0}
      mask prompts: fld "Fluid Type"; T_init "Initial Outlet Temperature [°C]"; Tamb_init "Initial Ambient Temperature [°C]"; f "Tube Friction Factor [-]"; KL_tube "Tube Minor Losses [-]"; KL "Total Minor Losses [-]"; H "Heat Transfer Coefficient [W/m²K]"; D "Pipe Internal Diameter [m]"; L "Pipe Length [m]"; t "Tube Wall Thickness [m]"; E "Tube Modulus of Elasticity [kPa]"; v "Tube Poisson Ratio [-]"; dH "Height between Inlet and Outlet [m]"; e_rough "Surface Roughness [m] (0.0015mm for copper, 0.01mm for rubber, 0mm for plastic)"; Num_MFRS "Number of Mass Flow Rate Sensors"; Num_PS "Number of Pressure Sensors"; Num_TS "Number of Temperature Sensors"; Num_BV "Number of Ball Valves"; Num_CV "Number of Check Valves"
      mask help: Models a pipe given upstream and downstream pressures.
      mask init:
      | load('Fluids.mat');
      | Fluid = eval(['Fluid.',fld]);
      | 
      | load('Moody.mat');
      | 
      | KL = KL_correction(KL_tube,Num_MFRS,Num_PS,Num_TS,Num_BV,Num_CV);
      | set_param(gcb,'KL',num2str(KL));
      settings: OpenFcn=|
      | load('Fluids.mat');
      | Set_Fluid_Popup_Names( Fluid )
      mask TypeOptions fld: Fuel | Water | Air | PG50
      mask DialogControl Container8 Prompt: Parameters
      mask DialogControl Container10 Prompt: Nonlinear Model
      mask DialogControl NomValuesGroupVar Prompt: Component Sizing - Nominal Values
      mask DialogControl Container11 Prompt: Linear Model
      mask DialogControl Container17 Prompt: Sensors and Valves
      mask Display:
      | if sum([Num_MFRS,Num_PS,Num_TS,Num_BV,Num_CV])==0
      |     image(imread('Tube.jpg'))
      | elseif sum([Num_MFRS,Num_PS,Num_TS])~=0 && sum([Num_BV,Num_CV])==0
      |     image(imread('Tube_Sensor.jpg'))
      | elseif sum([Num_MFRS,Num_PS,Num_TS])==0 && sum([Num_BV,Num_CV])~=0
      |     image(imread('Tube_Valve.jpg'))
      | else
      |     image(imread('Tube_Valve_Sensor.jpg'))
      | end
      | 
      | text(0.5,0.95,['{\bf ',fld,' Pipe (P to P)}'],'TexMode','on','horizontalAlignment', 'center')
      | text(0.5,0.1,['{-----}'],'TexMode','on','horizontalAlignment', 'center')
      | 
      | port_label('input',1,'Flow In')
      | port_label('input',2,'Amb. Temp. [°C]')
      | port_label('output',1,'Flow Out')
  Pump : Subsystem  mask(Centrifugal Pump){fld=PG50, P_init=145, T_init=22, H=0, D=13*1e-3, L=0.1, t=0.0015, E=2.4e6, v=0.4, A=1.27e-4, Rho_pump=1041, H_k=[-0.0767 9.33e-2 0.530], Eta_k=[6.717 18.75 -26.92 -0.0174 23 -22.89]}
      mask prompts: fld "Fluid Type"; P_init "Intial Outlet Pressure [kPa]"; T_init "Intial Outlet Temperature [°C]"; H "Heat Transfer Coefficient [W/m²K]"; D "Pipe Internal Diameter [m]"; L "Pipe Length [m]"; t "Tube Wall Thickness [m]"; E "Tube Modulus of Elasticity [kPa]"; v "Tube Poisson Ratio [-]"; A "Area used in pump head calculation [m²]"; Rho_pump "Density used in pump head calculation [kg/m³]"; H_k "Pump head map coefficients [K dP PWM]"; Eta_k "Pump efficiency coefficients [K WHP PWM WHP^2 PWM^2 WHP*PWM]"
      mask help: Tracks the time rate of change of fluid temperature, mass flow rate, and power consumption.
      mask init:
      | load('Fluids.mat');
      | Fluid = eval(['Fluid.',fld]);
      settings: OpenFcn=|
      | load('Fluids.mat');
      | Set_Fluid_Popup_Names( Fluid )
      mask TypeOptions fld: Fuel | Water | Air | PG50
      mask DialogControl Container11 Prompt: Parameters
      mask DialogControl Container14 Prompt: Nonlinear Model
      mask DialogControl Container15 Prompt: Component Sizing - Nominal Values
      mask DialogControl Container17 Prompt: Linear Model
      mask Display:
      | image(imread('Pump.jpg'))
      | 
      | text(0.5,0.95,['{\bf ',fld,' Pump}'],'TexMode','on','horizontalAlignment', 'center')
      | text(0.5,0.1,['{-----(P)}'],'TexMode','on','horizontalAlignment', 'center')
      | 
      | port_label('input',1,'Flow In')
      | port_label('input',2,'Duty Cycle [%]')
      | port_label('output',1,'Flow Out')
  Specify_Mass_Flow_Rate : Subsystem  mask(Flow Sink (Mass Flow Rate)){M_ext=on, M=0, T_ext=on, T=0, P_ext=on, P=0}
      mask prompts: M_ext "Mass flow rate time varying?"; M "Mass flow rate (kg/s)"; T_ext "Temperature time varying?"; T "Temperature (C)"; P_ext "Pressure time varying?"; P "Pressure (kPa)"
      mask help: Used to create a flow sink.
      mask Callback M_ext:
      | en = get_param(gcb,'MaskVisibilities');
      | h      = get_param(gcb,'handle');   % Get block handle
      | blk    = gcb;
      | hblock = get(h);     % Parse out handles structure
      | 
      | switch get_param(gcb,'M_ext')
      |     case 'on'
      |         en{2} = 'off';
      |         %add_block('simulink/Ports & Subsystems/In1',   [blk,'/In1'],'Position',[130    -7   160     7]);         % adding inport
      | 
      |     case 'off'
      |         en{2} = 'on';
      |         %delete_block([blk,'/In1'])
      | 
      | end
      | set_param(gcb,'MaskVisibilities',en);
      mask Callback T_ext:
      | en = get_param(gcb,'MaskVisibilities');
      | 
      | switch get_param(gcb,'T_ext')
      |     case 'on'
      |         en{4} = 'off';
      |     case 'off'
      |         en{4} = 'on';
      | end
      | set_param(gcb,'MaskVisibilities',en);
      mask Callback P_ext:
      | en = get_param(gcb,'MaskVisibilities');
      | 
      | switch get_param(gcb,'P_ext')
      |     case 'on'
      |         en{6} = 'off';
      |     case 'off'
      |         en{6} = 'on';
      | end
      | set_param(gcb,'MaskVisibilities',en);
      mask Display:
      | text(0.5,0.95,['{\bf Specify Mass Flow Rate}'],'TexMode','on','horizontalAlignment', 'center')
      | text(0.5,0.1,['{-----}'],'TexMode','on','horizontalAlignment', 'center')
      | 
      | port_label('input',1,'Flow In')
      | port_label('input',2,'Mass Flow Rate [kg/s]')
      | 
      | port_label('output',1,'Flow Out')
  Valve_P_to_M : Subsystem  mask(Continuous Valve (P to M)){fld=PG50, T_init=22, P_init=150, Tamb_init=22, f=0.05, KL=0, H=0, D=0.013, L=0.1, t=0.0015, E=2.4e6, v=0.4, e_rough=0.01*1e-3}
      mask prompts: fld "Fluid Type"; T_init "Initial Outlet Temperature [°C]"; P_init "Initial Outlet Pressure [kPa]"; Tamb_init "Initial Ambient Temperature [°C]"; f "Tube Friction Factor [-]"; KL "Minor Losses [-]"; H "Heat Transfer Coefficient [W/m²K]"; D "Internal Diameter [m]"; L "Length [m]"; t "Tube Wall Thickness [m]"; E "Tube Modulus of Elasticity [kPa]"; v "Tube Poisson Ratio [-]"; e_rough "Surface Roughness [m] (0.0015mm for copper, 0.01mm for rubber, 0mm for plastic)"
      mask help: Models a continuously variable valve given an upstream pressure and downstream mass flow rate.
      mask init:
      | load('Fluids.mat');
      | Fluid = eval(['Fluid.',fld]);
      | 
      | load('Moody.mat');
      settings: OpenFcn=|
      | load('Fluids.mat');
      | Set_Fluid_Popup_Names( Fluid )
      mask TypeOptions fld: Fuel | Water | Air | PG50
      mask DialogControl Container8 Prompt: Parameters
      mask DialogControl Container10 Prompt: Nonlinear Model
      mask DialogControl NomValuesGroupVar Prompt: Component Sizing - Nominal Values
      mask DialogControl Container11 Prompt: Linear Model
      mask Display:
      | image(imread('Solenoid.jpg'))
      | 
      | text(0.5,0.95,['{\bf ',fld,' Continuous Valve (P to M)}'],'TexMode','on','horizontalAlignment', 'center')
      | text(0.5,0.1,['{-----(P)}'],'TexMode','on','horizontalAlignment', 'center')
      | 
      | port_label('input',1,'Flow In')
      | port_label('input',2,'Fraction Open [0,1]')
      | port_label('output',1,'Flow Out')
  Valve_P_to_P : Subsystem  mask(Continuous Valve (P to P)){fld=PG50, T_init=22, f=0.05, KL=0, D=0.013, L=0.1}
      mask prompts: fld "Fluid Type"; T_init "Initial Outlet Temperature [°C]"; f "Friction Factor [-]"; KL "Minor Losses [-]"; D "Internal Diameter [m]"; L "Length [m]"
      mask help: Models a continuously variable valve given upstream and downstream pressures.
      mask init:
      | load('Fluids.mat');
      | Fluid = eval(['Fluid.',fld]);
      | 
      | load('Moody.mat');
      settings: OpenFcn=|
      | load('Fluids.mat');
      | Set_Fluid_Popup_Names( Fluid )
      mask TypeOptions fld: Fuel | Water | Air | PG50
      mask DialogControl Container8 Prompt: Parameters
      mask DialogControl Container10 Prompt: Nonlinear Model
      mask DialogControl NomValuesGroupVar Prompt: Component Sizing - Nominal Values
      mask DialogControl Container11 Prompt: Linear Model
      mask Display:
      | image(imread('Solenoid.jpg'))
      | 
      | 
      | text(0.5,0.95,['{\bf ',fld,' Continuous Valve (P to P)}'],'TexMode','on','horizontalAlignment', 'center')
      | text(0.5,0.1,['{-----}'],'TexMode','on','horizontalAlignment', 'center')
      | 
      | port_label('input',1,'Flow In')
      | port_label('input',2,'Fraction Open [0,1]')
      | port_label('output',1,'Flow Out')
